simulink subsystem "power_window_ECU"  (R2021a)
settings: Solver=VariableStepAuto  StartTime=0.0  StopTime=10.0  RelTol=1e-3
settings Model: Creator=achu  LastModifiedBy=Sai229

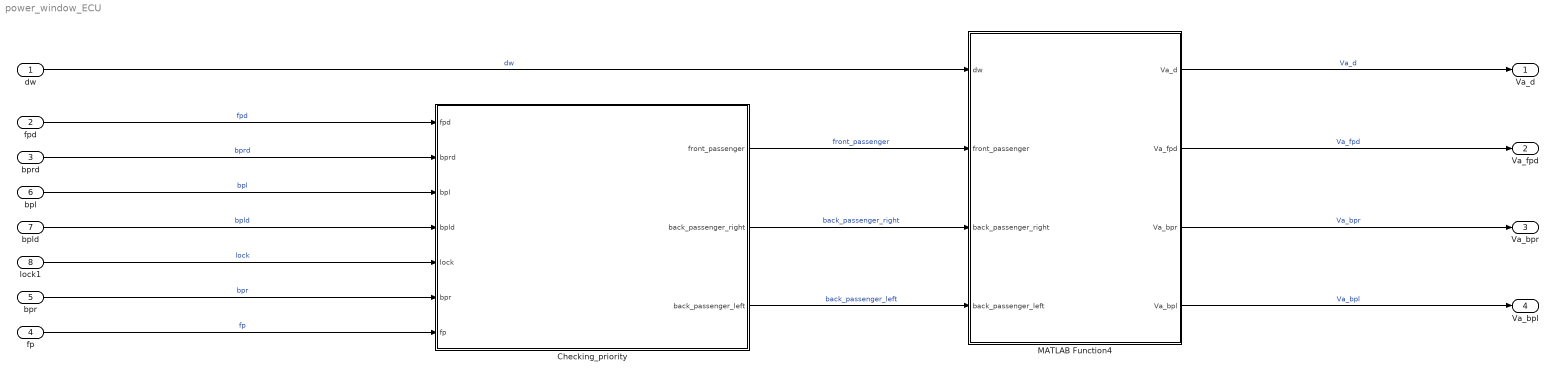
== system power_window_ECU ==
  dw : Inport
  fpd : Inport  Port=2
  bprd : Inport  Port=3
  fp : Inport  Port=4
  bpr : Inport  Port=5
  bpl : Inport  Port=6
  bpld : Inport  Port=7
  lock1 : Inport  Port=8
  Checking_priority : Subsystem  TreatAsAtomicUnit=on
  MATLAB Function4 : MATLAB Function  TreatAsAtomicUnit=on
  Va_d : Outport
  Va_fpd : Outport  Port=2
  Va_bpr : Outport  Port=3
  Va_bpl : Outport  Port=4
  wires:
  MATLAB Function4/2(Va_fpd) -> Va_fpd/1  "Va_fpd"
  MATLAB Function4/3(Va_bpr) -> Va_bpr/1  "Va_bpr"
  lock1/1 -> Checking_priority/5(lock)  "lock"
  fpd/1 -> Checking_priority/1(fpd)  "fpd"
  bpld/1 -> Checking_priority/4(bpld)  "bpld"
  MATLAB Function4/4(Va_bpl) -> Va_bpl/1  "Va_bpl"
  MATLAB Function4/1(Va_d) -> Va_d/1  "Va_d"
  Checking_priority/1(front_passenger) -> MATLAB Function4/2(front_passenger)  "front_passenger"
  dw/1 -> MATLAB Function4/1(dw)  "dw"
  bpl/1 -> Checking_priority/3(bpl)  "bpl"
  Checking_priority/2(back_passenger_right) -> MATLAB Function4/3(back_passenger_right)  "back_passenger_right"
  fp/1 -> Checking_priority/7(fp)  "fp"
  bpr/1 -> Checking_priority/6(bpr)  "bpr"
  bprd/1 -> Checking_priority/2(bprd)  "bprd"
  Checking_priority/3(back_passenger_left) -> MATLAB Function4/4(back_passenger_left)  "back_passenger_left"

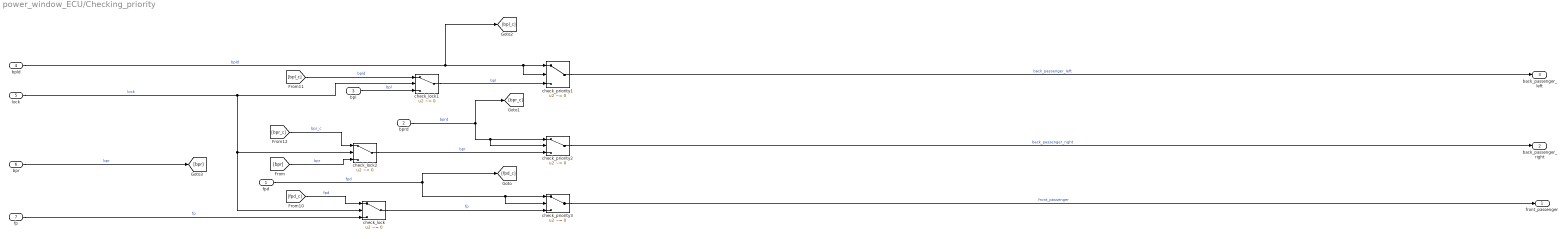
== system power_window_ECU/Checking_priority ==
  fpd : Inport
  bprd : Inport  Port=2
  bpl : Inport  Port=3
  bpld : Inport  Port=4
  lock : Inport  Port=5
  bpr : Inport  Port=6
  fp : Inport  Port=7
  check_lock : Switch  Criteria=u2 ~= 0
  check_lock1 : Switch  Criteria=u2 ~= 0
  check_lock2 : Switch  Criteria=u2 ~= 0
  check_priority1 : Switch  Criteria=u2 ~= 0
  check_priority2 : Switch  Criteria=u2 ~= 0
  check_priority3 : Switch  Criteria=u2 ~= 0
  front_passenger : Outport
  back_passenger_right : Outport  Port=2
  back_passenger_left : Outport  Port=3
  wires:
  fp/1 -> check_lock/3  "fp"
  bpr/1 -> [bpr]  "bpr"
  lock/1 -> check_lock1/2, check_lock2/2, check_lock/2  "lock"
  check_priority3/1 -> front_passenger/1  "front_passenger"
  check_priority2/1 -> back_passenger_right/1  "back_passenger_right"
  check_priority1/1 -> back_passenger_left/1  "back_passenger_left"
  bpld/1 -> check_priority1/2, check_priority1/1, [bpl_c]  "bpld"
  [bpr] -> check_lock2/3  "bpr"
  fpd/1 -> check_priority3/1, check_priority3/2, [fpd_c]  "fpd"
  bprd/1 -> [bpr_c], check_priority2/1, check_priority2/2  "bprd"
  [fpd_c] -> check_lock/1  "fpd"
  check_lock1/1 -> check_priority1/3  "bpl"
  [bpl_c] -> check_lock1/1  "bpld"
  check_lock2/1 -> check_priority2/3  "bpr"
  bpl/1 -> check_lock1/3  "bpl"
  [bpr_c] -> check_lock2/1  "bpr_c"
  check_lock/1 -> check_priority3/3  "fp"

== matlab function power_window_ECU/MATLAB Function4 ==
  data: dw input; Va_d output; front_passenger input; back_passenger_right input; back_passenger_left input; Va_fpd output; Va_bpr output; Va_bpl output
function [Va_d,Va_fpd, Va_bpr, Va_bpl] = fcn(dw, front_passenger, back_passenger_right, back_passenger_left)
dout=0;
fpd=0;
bpr=0;
bpl=0;
if (dw==1)
    dout=20;
elseif (dw==-1)
    dout=-20;
elseif (dw==0)
    dout=0;
end

if (front_passenger==1)
        fpd=20;
elseif (front_passenger==-1)
    fpd=-20;
elseif (front_passenger==0)
    fpd=0;
end

if (back_passenger_right==1)
        bpr=20;
elseif (back_passenger_right==-1)
    bpr=-20;
elseif (back_passenger_right==0)
    bpr=0;
end

if (back_passenger_left==1)
        bpl=20;
elseif (back_passenger_left==-1)
    bpl=-20;
elseif (back_passenger_left==0)
    bpl=0;
end
  
Va_d = dout;
Va_fpd = fpd;
Va_bpr=bpr;
Va_bpl=bpl;
